simulink model "lateral control"  (R2020a)
settings: Solver=VariableStepAuto  StartTime=0.0  StopTime=60  RelTol=1e-3
libraries: Solver_SF x1
settings Model: Creator=hello1996hello  LastModifiedBy=hello1996hello
settings DataIOCC: ReturnWorkspaceOutputs=off

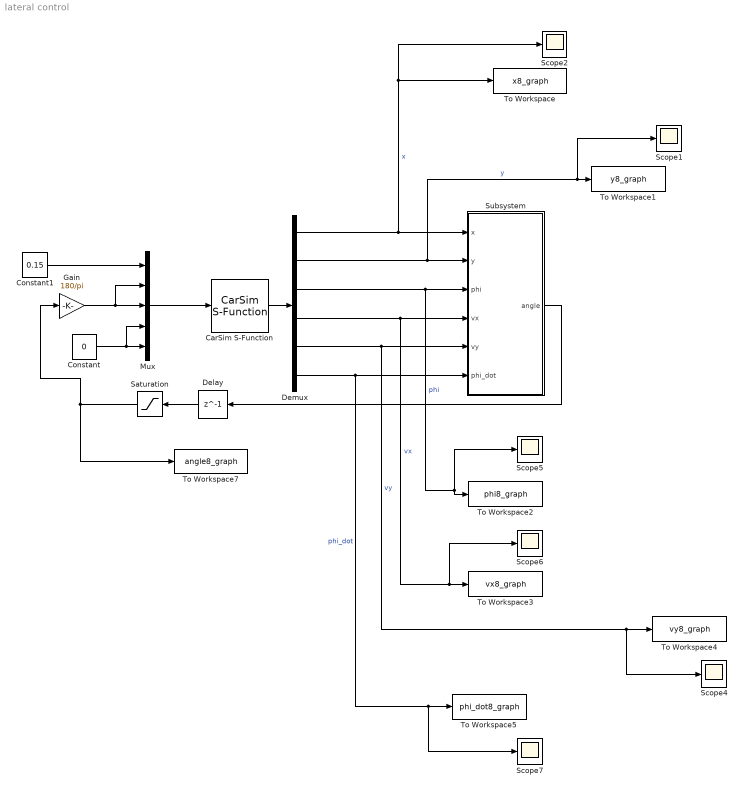
== system lateral control ==
  CarSim S-Function : Solver_SF/CarSim S-Function  Priority=1  SIMFILE=simfile.sim  Run_RTs=off  vs_state_ind=Run  StopMode_ind=Vehicle Model
  Constant : Constant  Value=0
  Constant1 : Constant  Value=0.15
  Delay : Delay  DelayLength=1  UseCircularBuffer=on
  Demux : Demux  Outputs=6
  Gain : Gain  Gain=180/pi
  Mux : Mux  Inputs=5
  Saturation : Saturate  UpperLimit=1.2  LowerLimit=-1.2
  Scope{1..2,4..7} (6 alike) : Scope
  Subsystem : Subsystem
  To Workspace : ToWorkspace  VariableName=x8_graph  SaveFormat=Timeseries  SampleTime=-1
  To Workspace1 : ToWorkspace  VariableName=y8_graph  SaveFormat=Timeseries  SampleTime=-1
  To Workspace2 : ToWorkspace  VariableName=phi8_graph  SaveFormat=Timeseries  SampleTime=-1
  To Workspace3 : ToWorkspace  VariableName=vx8_graph  SaveFormat=Timeseries  SampleTime=-1
  To Workspace4 : ToWorkspace  VariableName=vy8_graph  SaveFormat=Timeseries  SampleTime=-1
  To Workspace5 : ToWorkspace  VariableName=phi_dot8_graph  SaveFormat=Timeseries  SampleTime=-1
  To Workspace7 : ToWorkspace  VariableName=angle8_graph  SaveFormat=Timeseries  SampleTime=-1
  wires:
  Delay/1 -> Saturation/1
  Demux/1 -> Scope2/1, To Workspace/1, Subsystem/1(x)  "x"
  Constant1/1 -> Mux/1
  CarSim S-Function/1 -> Demux/1
  Constant/1 -> Mux/4, Mux/5
  Demux/4 -> Scope6/1, To Workspace3/1, Subsystem/4(vx)  "vx"
  Demux/6 -> Scope7/1, To Workspace5/1, Subsystem/6(phi_dot)  "phi_dot"
  Demux/5 -> Scope4/1, To Workspace4/1, Subsystem/5(vy)  "vy"
  Demux/3 -> Scope5/1, To Workspace2/1, Subsystem/3(phi)  "phi"
  Demux/2 -> Scope1/1, To Workspace1/1, Subsystem/2(y)  "y"
  Subsystem/1(angle) -> Delay/1
  Mux/1 -> CarSim S-Function/1
  Saturation/1 -> To Workspace7/1, Gain/1
  Gain/1 -> Mux/2, Mux/3

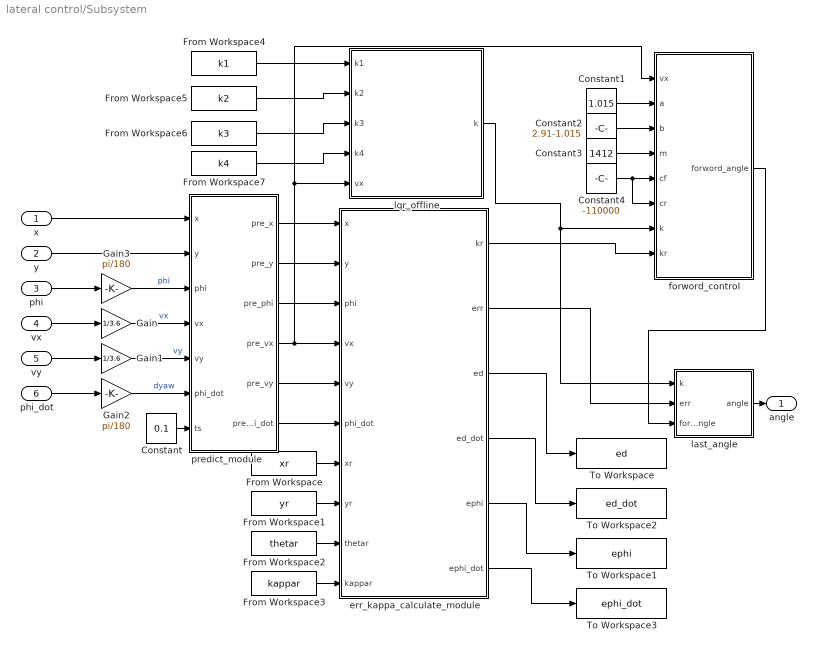
== system lateral control/Subsystem ==
  x : Inport
  y : Inport  Port=2
  phi : Inport  Port=3
  vx : Inport  Port=4
  vy : Inport  Port=5
  phi_dot : Inport  Port=6
  Constant : Constant  Value=0.1
  Constant1 : Constant  Value=1.015
  Constant2 : Constant  Value=2.91-1.015
  Constant3 : Constant  Value=1412
  Constant4 : Constant  Value=-110000
  From Workspace : FromWorkspace  VariableName=xr
  From Workspace1 : FromWorkspace  VariableName=yr
  From Workspace2 : FromWorkspace  VariableName=thetar
  From Workspace3 : FromWorkspace  VariableName=kappar
  From Workspace4 : FromWorkspace  VariableName=k1
  From Workspace5 : FromWorkspace  VariableName=k2
  From Workspace6 : FromWorkspace  VariableName=k3
  From Workspace7 : FromWorkspace  VariableName=k4
  Gain : Gain  Gain=1/3.6
  Gain1 : Gain  Gain=1/3.6
  Gain2 : Gain  Gain=pi/180
  Gain3 : Gain  Gain=pi/180
  To Workspace : ToWorkspace  VariableName=ed  SaveFormat=Timeseries  SampleTime=-1
  To Workspace1 : ToWorkspace  VariableName=ephi  SaveFormat=Timeseries  SampleTime=-1
  To Workspace2 : ToWorkspace  VariableName=ed_dot  SaveFormat=Timeseries  SampleTime=-1
  To Workspace3 : ToWorkspace  VariableName=ephi_dot  SaveFormat=Timeseries  SampleTime=-1
  err_kappa_calculate_module : MATLAB Function  TreatAsAtomicUnit=on
  forword_control : MATLAB Function  TreatAsAtomicUnit=on
  last_angle : MATLAB Function  TreatAsAtomicUnit=on
  lqr_offline : MATLAB Function  TreatAsAtomicUnit=on
  predict_module : MATLAB Function  TreatAsAtomicUnit=on
  angle : Outport  VectorParamsAs1DForOutWhenUnconnected=off
  wires:
  From Workspace7/1 -> lqr_offline/4(k4)
  err_kappa_calculate_module/2(err) -> last_angle/2(err)
  Gain1/1 -> predict_module/5(vy)  "vy"
  From Workspace6/1 -> lqr_offline/3(k3)
  x/1 -> predict_module/1(x)
  lqr_offline/1(k) -> last_angle/1(k), forword_control/7(k)
  phi_dot/1 -> Gain2/1
  predict_module/2(pre_y) -> err_kappa_calculate_module/2(y)
  err_kappa_calculate_module/1(kr) -> forword_control/8(kr)
  forword_control/1(forword_angle) -> last_angle/3(forword_angle)
  vx/1 -> Gain/1
  predict_module/4(pre_vx) -> lqr_offline/5(vx), forword_control/1(vx), err_kappa_calculate_module/4(vx)
  Gain2/1 -> predict_module/6(phi_dot)  "dyaw"
  last_angle/1(angle) -> angle/1
  phi/1 -> Gain3/1
  From Workspace2/1 -> err_kappa_calculate_module/9(thetar)
  From Workspace5/1 -> lqr_offline/2(k2)
  Gain/1 -> predict_module/4(vx)  "vx"
  y/1 -> predict_module/2(y)
  Gain3/1 -> predict_module/3(phi)  "phi"
  From Workspace3/1 -> err_kappa_calculate_module/10(kappar)
  Constant/1 -> predict_module/7(ts)
  From Workspace4/1 -> lqr_offline/1(k1)
  From Workspace1/1 -> err_kappa_calculate_module/8(yr)
  predict_module/1(pre_x) -> err_kappa_calculate_module/1(x)
  predict_module/5(pre_vy) -> err_kappa_calculate_module/5(vy)
  vy/1 -> Gain1/1
  From Workspace/1 -> err_kappa_calculate_module/7(xr)
  predict_module/6(pre_phi_dot) -> err_kappa_calculate_module/6(phi_dot)
  predict_module/3(pre_phi) -> err_kappa_calculate_module/3(phi)
  Constant1/1 -> forword_control/2(a)
  Constant2/1 -> forword_control/3(b)
  Constant3/1 -> forword_control/4(m)
  Constant4/1 -> forword_control/6(cr), forword_control/5(cf)
  err_kappa_calculate_module/3(ed) -> To Workspace/1
  err_kappa_calculate_module/4(ed_dot) -> To Workspace2/1
  err_kappa_calculate_module/5(ephi) -> To Workspace1/1
  err_kappa_calculate_module/6(ephi_dot) -> To Workspace3/1

== matlab function lateral control/Subsystem/err_kappa_calculate_module ==
  data: x input; kr output; y input; phi input; vx input; vy input; phi_dot input; xr input; yr input; thetar input; kappar input; err output; ed output; ed_dot output; ephi output; ephi_dot output
function [kr,err,ed,ed_dot,ephi,ephi_dot] = fcn(x,y,phi,vx,vy,phi_dot,xr,yr,thetar,kappar)
    n=length(xr);%数组中点的个数
    d_min=(x-xr(1))^2+(y-yr(1))^2;
    min=1;
    for i=1:n
        d=(x-xr(i))^2+(y-yr(i))^2;
        if d<d_min
            d_min=d;
            min=i;
        end

    end
    dmin=min;
    
 %%%%%%%%%%%%%%%%%%%%%%%%%%%%%%%%%%%%%%%%%%%修改LQR%%%%%%%%%%%%%%%%%%%%%%%%%%%%%%%   
%     if ((dmin>=1)&&(dmin<=200))||((dmin>=601)&&(dmin<=800))||((dmin>=1001)&&(dmin<=1200))||((dmin>=1401)&&(dmin<=1600))||((dmin>=1801)&&(dmin<=2000))||((dmin>=2401)&&(dmin<=2599))
%         projection_point_thetar=thetar(dmin); 
%     elseif ((dmin>=401)&&(dmin<=600))||((dmin>=1201)&&(dmin<=1400))||((dmin>=2001)&&(dmin<=2200))
%         projection_point_thetar=thetar(dmin)+1.858*3.14/180;
%     else
%         projection_point_thetar=thetar(dmin)-1.858*3.14/180;
%     end
 %%%%%%%%%%%%%%%%%%%%%%%%%%%%%%%%%%%%%%%%%%%%%%%%%%%%%%%%%%%%%%%%%%%%%%%%%%%%%%%%%%%%%%
 
   
%     if ((dmin>=1)&&(dmin<=400))||((dmin>=1201)&&(dmin<=1600))||((dmin>=2001)&&(dmin<=2400))||((dmin>=2801)&&(dmin<=3200))||((dmin>=3601)&&(dmin<=4000))||((dmin>=4801)&&(dmin<=5199))
%         projection_point_thetar=thetar(dmin); 
%     elseif ((dmin>=801)&&(dmin<=1200))||((dmin>=2401)&&(dmin<=2800))||((dmin>=4001)&&(dmin<=4400))
%         projection_point_thetar=thetar(dmin)+1.858*3.14/180;
%     else
%         projection_point_thetar=thetar(dmin)-1.858*3.14/180;
%     end
 %%%%%%%%%%%%%%%%%%%%%%%%%%%%%%%%%%%%%%%%%%%%%%%%%%%%%%%%%%%%%%%%%%%%%%%%%%%%%%%%%%%%%%
 

%     if (dmin>1)&&(dmin<2599)
%         d1=(x-xr(dmin-1))^2+(y-yr(dmin-1))^2;
%         d2=(x-xr(dmin+1))^2+(y-yr(dmin+1))^2;
%         if d1<d2
%             projection_point_thetar=thetar(dmin)-1.858*3.14/180; 
%         else
%             projection_point_thetar=thetar(dmin)+1.858*3.14/180;
%         end
%     else
%         projection_point_thetar=thetar(dmin); 
%     end

    %%%%%%%%%%%%%%%%%%%%%%%%%%%%%%%%%%%%%%%%%%%%%%%%%%%%%%%%%%%%%%%%%%%%%%%%%%%%%%%%%

    
    
    
    tor=[cos(thetar(dmin));sin(thetar(dmin))];
    nor=[-sin(thetar(dmin));cos(thetar(dmin))];
    d_err=[x-xr(dmin);y-yr(dmin)];
    ed=nor'*d_err;
    es=tor'*d_err;
    

    projection_point_thetar=thetar(dmin)+1.858*3.14/180; %  DT function
    
   

    ed_dot=vy*cos(phi-projection_point_thetar)+vx*sin(phi-projection_point_thetar);
    %%%%%%%%%
    ephi=sin(phi-projection_point_thetar);
    %%%%%%%%%
    s_dot=vx*cos(phi-projection_point_thetar)-vy*sin(phi-projection_point_thetar);
    s_dot=s_dot/(1-kappar(dmin)*ed);
    ephi_dot=phi_dot-kappar(dmin)*s_dot;
    kr=kappar(dmin);
    err=[ed;ed_dot;ephi;ephi_dot];
    
end

== matlab function lateral control/Subsystem/predict_module ==
  data: x input; pre_x output; y input; phi input; vx input; vy input; phi_dot input; ts input; pre_y output; pre_phi output; pre_vx output; pre_vy output; pre_phi_dot output
function [pre_x,pre_y,pre_phi,pre_vx,pre_vy,pre_phi_dot] = fcn(x,y,phi,vx,vy,phi_dot,ts)
    pre_x=x+vx*ts*cos(phi)-vy*ts*sin(phi);
    pre_y=y+vy*ts*cos(phi)+vx*ts*sin(phi);
    pre_phi=phi+phi_dot*ts;
    pre_vx=vx;
    pre_vy=vy;
    pre_phi_dot=phi_dot;
end

== matlab function lateral control/Subsystem/lqr_offline ==
  data: k1 input; k output; k2 input; k3 input; k4 input; vx input
function k  = fcn(k1,k2,k3,k4,vx)
    if abs(vx)<0.01
        k=[0,0,0,0];
    else
        index=round(vx/0.01);
        k=[k1(index),k2(index),k3(index),k4(index)];
    end
end

== matlab function lateral control/Subsystem/forword_control ==
  data: vx input; a input; forword_angle output; b input; m input; cf input; cr input; k input; kr input
function forword_angle = fcn(vx,a,b,m,cf,cr,k,kr)
    forword_angle=kr*(a+b-b*k(3)-(m*vx*vx/(a+b))*((b/cf)+(a/cr)*k(3)-(a/cr)));
end

== matlab function lateral control/Subsystem/last_angle ==
  data: k input; angle output; err input; forword_angle input
function angle = fcn(k,err,forword_angle)

    angle=-k*err+forword_angle;
end
